simulink model "partD"  (R2018b)
settings: Solver=VariableStepAuto  StartTime=0.0  StopTime=10.0  RelTol=1e-3
settings Model: Creator=amir  LastModifiedBy=amir

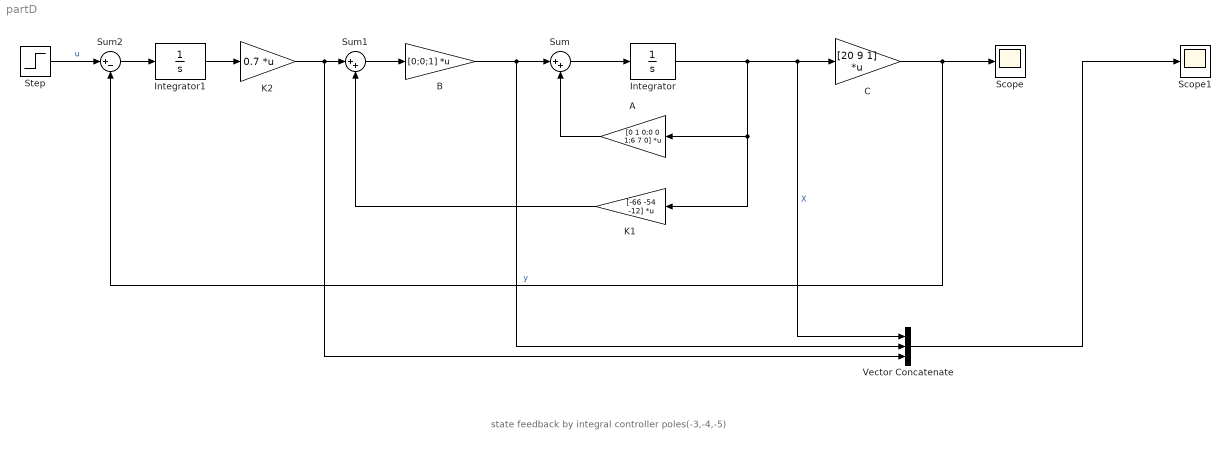
== system partD ==
  note: state feedback by integral controller
      | poles(-3,-4,-5)
  A : Gain  Gain=[0 1 0;0 0 1;6 7 0]  Multiplication=Matrix(K*u) (u vector)
  B : Gain  Gain=[0;0;1]  Multiplication=Matrix(K*u) (u vector)
  C : Gain  Gain=[20 9 1]  Multiplication=Matrix(K*u) (u vector)
  Integrator : Integrator  InitialCondition=[1;1;1]
  Integrator1 : Integrator  InitialCondition=[1]
  K1 : Gain  Gain=[-66 -54 -12]  Multiplication=Matrix(K*u) (u vector)
  K2 : Gain  Gain=0.7  Multiplication=Matrix(K*u) (u vector)
  Scope : Scope
  Scope1 : Scope
  Step : Step  After=5  SampleTime=0
  Sum : Sum  Inputs=|++
  Sum1 : Sum  Inputs=|++
  Sum2 : Sum  Inputs=|+-
  Vector Concatenate : Concatenate  NumInputs=3
  wires:
  B/1 -> Vector Concatenate/2, Sum/1
  Sum/1 -> Integrator/1
  Integrator/1 -> A/1, K1/1, Vector Concatenate/1, C/1  "X"
  C/1 -> Sum2/2, Scope/1  "y"
  A/1 -> Sum/2
  Sum1/1 -> B/1
  K1/1 -> Sum1/2
  K2/1 -> Vector Concatenate/3, Sum1/1
  Integrator1/1 -> K2/1
  Sum2/1 -> Integrator1/1
  Step/1 -> Sum2/1  "u"
  Vector Concatenate/1 -> Scope1/1
